simulink subsystem "D1Szakaszteljes"  (R2024b)
settings: Solver=VariableStepAuto  StartTime=0.0  StopTime=10.0  RelTol=1e-3
undefined symbols (not defined in the file or in its folder): R
settings Model: Creator=Asus  LastModifiedBy=Asus

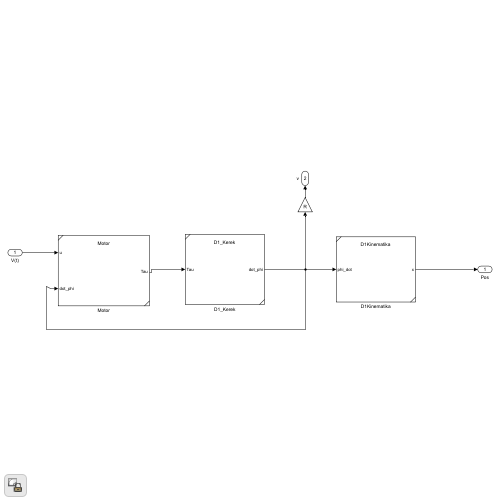
[thumbnail: Simulink's stored preview of the top-level diagram]
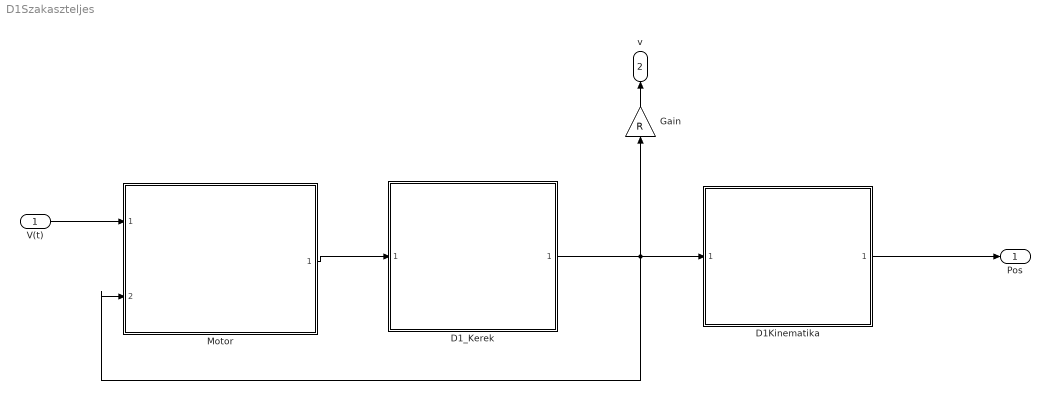
== system D1Szakaszteljes ==
  V(t) : Inport
  D1Kinematika : Subsystem  ReferencedSubsystem=D1Kinematika
  D1_Kerek : Subsystem  ReferencedSubsystem=D1_Kerek
  Gain : Gain  Gain=R
  Motor : Subsystem  ReferencedSubsystem=Motor
  Pos : Outport
  v : Outport  Port=2
  wires:
  V(t)/1 -> Motor/1
  D1Kinematika/1 -> Pos/1
  Motor/1 -> D1_Kerek/1
  D1_Kerek/1 -> Motor/2, Gain/1, D1Kinematika/1
  Gain/1 -> v/1
